simulink model "sampleModel1864"  (R2023a)
settings: Solver=VariableStepAuto  StartTime=0.0  StopTime=10.0  RelTol=1e-3
libraries: hdlsllib x8, simulink x2
settings Model: Creator=user1  LastModifiedBy=user1

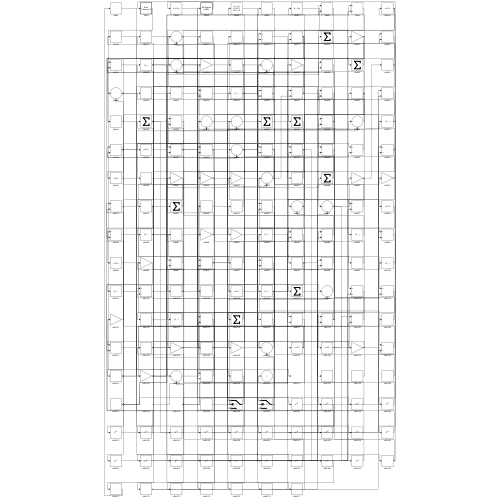
[thumbnail: Simulink's stored preview of the top-level diagram]
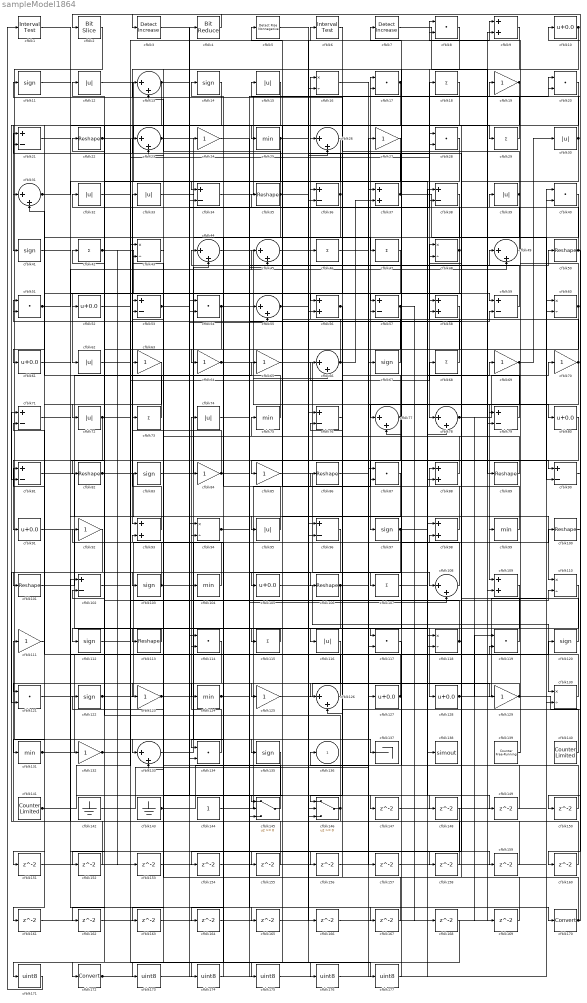
== system sampleModel1864 ==
  cfblk1 : hdlsllib/Logic and Bit Operations/Interval Test  IntervalClosedRight=on  uplimit=0.5  IntervalClosedLeft=on  lowlimit=-0.5  OutDataTypeStr=boolean
  cfblk{10,52,61,80,91,105,127..128} (8 alike) : Bias  Bias=0.0  SaturateOnIntegerOverflow=off
  cfblk{22,35,50,82,86,89,100..101,106,113} (10 alike) : Reshape
  cfblk{21,34,36,38,53,57,59,71,76,79,81,90,96,102} (14 alike) : Sum  Inputs=+-
  cfblk{11,14,41,67,83,97,103,112,120,122,135} (11 alike) : Signum
  cfblk{25,75,99,104,124,131} (6 alike) : MinMax
  cfblk{18,29,42,46..47,68,73,107,115} (9 alike) : Sum  Inputs=+
  cfblk{13,23,26,31,44..45,49,55,66,77..78,108,126,133} (14 alike) : Sum  Inputs=|++
  cfblk{9,37,56,58,88,93,98,109} (8 alike) : Sum
  cfblk{16,43,48,60,94,110,118,130} (8 alike) : Product  Inputs=*/  RndMeth=Zero  SaturateOnIntegerOverflow=on
  cfblk{19,24,27,63..65,69..70,84..85,92,111,123,125,129,132} (16 alike) : Gain
  cfblk{8,17,20,28,40,51,54,87,114,117,119,121,134} (13 alike) : DotProduct  OutDataTypeStr=Inherit: Inherit via internal rule
  cfblk{12,15,30,32..33,39,62,72,74,95,116} (11 alike) : Abs  SaturateOnIntegerOverflow=off
  cfblk137 : Terminator
  cfblk138 : ToWorkspace  VariableName=simout  SaveFormat=Timeseries  SampleTime=-1
  cfblk139 : hdlsllib/Sources/Counter Free-Running  NumBits=16  tsamp=-1
  cfblk140 : hdlsllib/Sources/Counter Limited  uplimit=7  tsamp=-1
  cfblk141 : hdlsllib/Sources/Counter Limited  uplimit=7  tsamp=-1
  cfblk142 : Ground
  cfblk143 : Ground
  cfblk144 : Constant  SampleTime=-1
  cfblk145 : Switch  SaturateOnIntegerOverflow=off  InputSameDT=off
  cfblk146 : Switch  SaturateOnIntegerOverflow=off  InputSameDT=off
  cfblk{147..169} (23 alike) : Delay  SampleTime=1
  cfblk170 : DataTypeConversion  SaturateOnIntegerOverflow=off  RndMeth=Floor
  cfblk{171,173..177} (6 alike) : DataTypeConversion  OutDataTypeStr=uint8  SaturateOnIntegerOverflow=off  RndMeth=Floor
  cfblk172 : DataTypeConversion  SaturateOnIntegerOverflow=off  RndMeth=Floor
  cfblk2 : hdlsllib/Logic and Bit Operations/Bit Slice  lidx=7  ridx=0
  cfblk3 : simulink/Logic and Bit Operations/Detect Increase  vinit=0.0  OutDataTypeStr=boolean
      settings: LibrarySourceBlock=|
      | hdlsllib/Logic and Bit
      | Operations/Detect
      | Increase
  cfblk4 : hdlsllib/Logic and Bit Operations/Bit Reduce  mode=AND
  cfblk5 : hdlsllib/Logic and Bit Operations/Detect Rise Nonnegative  vinit=0  OutDataTypeStr=boolean
  cfblk6 : hdlsllib/Logic and Bit Operations/Interval Test  IntervalClosedRight=on  uplimit=0.5  IntervalClosedLeft=on  lowlimit=-0.5  OutDataTypeStr=boolean
  cfblk7 : simulink/Logic and Bit Operations/Detect Increase  vinit=0.0  OutDataTypeStr=boolean
      settings: LibrarySourceBlock=|
      | hdlsllib/Logic and Bit
      | Operations/Detect
      | Increase
  cfblk136 : Outport  VectorParamsAs1DForOutWhenUnconnected=off
  wires:
  cfblk66/1 -> cfblk16/1, cfblk37/2
  cfblk23/1 -> cfblk137/1, cfblk36/2
  cfblk91/1 -> cfblk116/1
  cfblk117/1 -> cfblk136/1
  cfblk10/1 -> cfblk93/1, cfblk23/2
  cfblk2/1 -> cfblk133/1
  cfblk9/1 -> cfblk78/1
  cfblk56/1 -> cfblk85/1, cfblk146/1
  cfblk82/1 -> cfblk110/1, cfblk65/1
  cfblk105/1 -> cfblk130/1
  cfblk67/1 -> cfblk44/1
  cfblk85/1 -> cfblk107/1
  cfblk98/1 -> cfblk88/1
  cfblk14/1 -> cfblk41/1
  cfblk34/1 -> cfblk19/1
  cfblk47/1 -> cfblk62/1
  cfblk144/1 -> cfblk17/1
  cfblk131/1 -> cfblk120/1, cfblk119/2
  cfblk124/1 -> cfblk108/2, cfblk167/1
  cfblk26/1 -> cfblk115/1
  cfblk61/1 -> cfblk135/1
  cfblk103/1 -> cfblk22/1, cfblk38/2
  cfblk113/1 -> cfblk112/1
  cfblk83/1 -> cfblk44/2
  cfblk134/1 -> cfblk74/1
  cfblk48/1 -> cfblk18/1, cfblk61/1
  cfblk127/1 -> cfblk12/1, cfblk73/1
  cfblk122/1 -> cfblk100/1, cfblk134/2
  cfblk143/1 -> cfblk46/1, cfblk27/1
  cfblk120/1 -> cfblk51/1
  cfblk142/1 -> cfblk127/1
  cfblk42/1 -> cfblk94/1, cfblk153/1
  cfblk6/1 -> cfblk56/1
  cfblk51/1 -> cfblk132/1, cfblk49/2
  cfblk133/1 -> cfblk98/2
  cfblk146/1 -> cfblk111/1, cfblk102/2
  cfblk36/1 -> cfblk26/1, cfblk154/1
  cfblk84/1 -> cfblk49/1, cfblk43/2
  cfblk78/1 -> cfblk70/1, cfblk169/1
  cfblk59/1 -> cfblk11/1
  cfblk70/1 -> cfblk109/1, cfblk57/2
  cfblk54/1 -> cfblk64/1, cfblk20/2
  cfblk20/1 -> cfblk31/1
  cfblk116/1 -> cfblk121/1
  cfblk68/1 -> cfblk48/1
  cfblk72/1 -> cfblk91/1, cfblk8/1
  cfblk13/1 -> cfblk104/1, cfblk81/2
  cfblk69/1 -> cfblk30/1, cfblk117/2
  cfblk129/1 -> cfblk3/1, cfblk123/1
  cfblk21/1 -> cfblk56/2
  cfblk101/1 -> cfblk4/1
  cfblk89/1 -> cfblk75/1
  cfblk74/1 -> cfblk50/1
  cfblk50/1 -> cfblk32/1, cfblk160/1
  cfblk93/1 -> cfblk33/1
  cfblk111/1 -> cfblk81/1
  cfblk28/1 -> cfblk52/1
  cfblk44/1 -> cfblk80/1
  cfblk29/1 -> cfblk17/2
  cfblk75/1 -> cfblk63/1
  cfblk81/1 -> cfblk95/1
  cfblk8/1 -> cfblk57/1
  cfblk139/1 -> cfblk39/1
  cfblk11/1 -> cfblk25/1
  cfblk79/1 -> cfblk21/1
  cfblk112/1 -> cfblk83/1
  cfblk128/1 -> cfblk60/1, cfblk119/1
  cfblk115/1 -> cfblk113/1
  cfblk108/1 -> cfblk7/1
  cfblk57/1 -> cfblk82/1, cfblk168/1
  cfblk77/1 -> cfblk51/2, cfblk96/2
  cfblk114/1 -> cfblk172/1
  cfblk109/1 -> cfblk128/1
  cfblk118/1 -> cfblk42/1, cfblk48/2
  cfblk12/1 -> cfblk138/1
  cfblk31/1 -> cfblk34/1, cfblk156/1
  cfblk73/1 -> cfblk31/2
  cfblk39/1 -> cfblk77/1, cfblk146/3, cfblk13/1
  cfblk16/1 -> cfblk79/1
  cfblk132/1 -> cfblk110/2, cfblk28/1, cfblk165/1
  cfblk7/1 -> cfblk89/1
  cfblk41/1 -> cfblk90/1
  cfblk19/1 -> cfblk105/1, cfblk158/1
  cfblk125/1 -> cfblk129/1
  cfblk37/1 -> cfblk90/2, cfblk23/1
  cfblk17/1 -> cfblk117/1, cfblk151/1, cfblk152/1
  cfblk94/1 -> cfblk106/1, cfblk59/2
  cfblk102/1 -> cfblk43/1
  cfblk130/1 -> cfblk86/1
  cfblk60/1 -> cfblk8/2, cfblk173/1
  cfblk22/1 -> cfblk29/1, cfblk118/2
  cfblk38/1 -> cfblk77/2
  cfblk140/1 -> cfblk36/1
  cfblk141/1 -> cfblk6/1, cfblk146/2, cfblk68/1
  cfblk95/1 -> cfblk14/1
  cfblk97/1 -> cfblk69/1, cfblk131/1
  cfblk76/1 -> cfblk126/1
  cfblk46/1 -> cfblk67/1
  cfblk40/1 -> cfblk101/1
  cfblk65/1 -> cfblk97/1
  cfblk30/1 -> cfblk15/1, cfblk58/1
  cfblk32/1 -> cfblk59/1
  cfblk5/1 -> cfblk47/1
  cfblk25/1 -> cfblk34/2, cfblk159/1
  cfblk126/1 -> cfblk71/2
  cfblk33/1 -> cfblk76/1
  cfblk55/1 -> cfblk125/1, cfblk26/2, cfblk177/1
  cfblk49/1 -> cfblk5/1
  cfblk53/1 -> cfblk24/1, cfblk55/2
  cfblk99/1 -> cfblk35/1
  cfblk64/1 -> cfblk66/2, cfblk124/1
  cfblk119/1 -> cfblk21/2
  cfblk123/1 -> cfblk54/2, cfblk96/1
  cfblk43/1 -> cfblk103/1
  cfblk100/1 -> cfblk20/1
  cfblk1/1 -> cfblk170/1
  cfblk106/1 -> cfblk37/1, cfblk145/2, cfblk108/1
  cfblk4/1 -> cfblk2/1
  cfblk104/1 -> cfblk92/1
  cfblk58/1 -> cfblk134/1
  cfblk15/1 -> cfblk53/1
  cfblk88/1 -> cfblk53/2
  cfblk35/1 -> cfblk9/1, cfblk28/2, cfblk145/3, cfblk13/2
  cfblk27/1 -> cfblk72/1
  cfblk71/1 -> cfblk99/1
  cfblk121/1 -> cfblk84/1
  cfblk52/1 -> cfblk45/1
  cfblk92/1 -> cfblk121/2
  cfblk96/1 -> cfblk145/1
  cfblk145/1 -> cfblk122/1
  cfblk24/1 -> cfblk147/1
  cfblk147/1 -> cfblk40/2
  cfblk3/1 -> cfblk148/1
  cfblk107/1 -> cfblk149/1
  cfblk149/1 -> cfblk66/1
  cfblk90/1 -> cfblk150/1
  cfblk150/1 -> cfblk98/1
  cfblk151/1 -> cfblk55/1
  cfblk152/1 -> cfblk102/1
  cfblk153/1 -> cfblk133/2
  cfblk154/1 -> cfblk78/2
  cfblk80/1 -> cfblk155/1
  cfblk155/1 -> cfblk71/1
  cfblk156/1 -> cfblk60/2
  cfblk86/1 -> cfblk157/1
  cfblk157/1 -> cfblk130/2
  cfblk158/1 -> cfblk126/2
  cfblk159/1 -> cfblk54/1
  cfblk160/1 -> cfblk94/2
  cfblk63/1 -> cfblk161/1
  cfblk161/1 -> cfblk79/2
  cfblk18/1 -> cfblk162/1
  cfblk162/1 -> cfblk16/2
  cfblk135/1 -> cfblk163/1
  cfblk163/1 -> cfblk88/2
  cfblk110/1 -> cfblk164/1
  cfblk164/1 -> cfblk109/2
  cfblk165/1 -> cfblk9/2
  cfblk45/1 -> cfblk166/1
  cfblk166/1 -> cfblk38/1
  cfblk167/1 -> cfblk93/2
  cfblk169/1 -> cfblk76/2
  cfblk170/1 -> cfblk58/2, cfblk10/1
  cfblk168/1 -> cfblk171/1
  cfblk171/1 -> cfblk1/1
  cfblk172/1 -> cfblk45/2, cfblk40/1
  cfblk173/1 -> cfblk114/1
  cfblk148/1 -> cfblk174/1
  cfblk174/1 -> cfblk114/2
  cfblk87/1 -> cfblk175/1
  cfblk175/1 -> cfblk118/1
  cfblk62/1 -> cfblk176/1
  cfblk176/1 -> cfblk87/1
  cfblk177/1 -> cfblk87/2
